simulink model "practice1_sim"  (R2020b)
settings: Solver=FixedStepAuto  StartTime=0.0  StopTime=simtime  FixedStep=step  RelTol=1e-3
undefined symbols (not defined in the file or in its folder): D, JL, JM, K, KE, KT, L, La, Ra
settings Model: Creator=yuto  LastModifiedBy=yuto

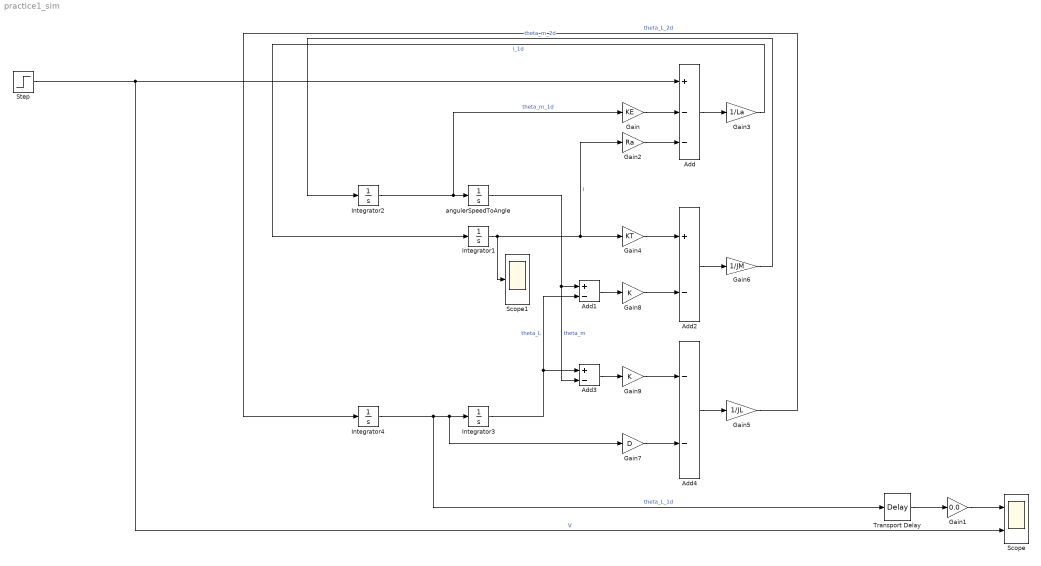
== system practice1_sim ==
  Add : Sum  Inputs=+--
  Add1 : Sum  Inputs=+-
  Add2 : Sum  Inputs=+-
  Add3 : Sum  Inputs=+-
  Add4 : Sum  Inputs=--
  Gain : Gain  Gain=KE
  Gain1 : Gain  Gain=0.0
  Gain2 : Gain  Gain=Ra
  Gain3 : Gain  Gain=1/La
  Gain4 : Gain  Gain=KT
  Gain5 : Gain  Gain=1/JL
  Gain6 : Gain  Gain=1/JM
  Gain7 : Gain  Gain=D
  Gain8 : Gain  Gain=K
  Gain9 : Gain  Gain=K
  Integrator{1..4} (4 alike) : Integrator
  Scope : Scope  NumInputPorts=2
  Scope1 : Scope
  Step : Step  Time=0  SampleTime=0
  Transport Delay : TransportDelay  DelayTime=L
  angulerSpeedToAngle : Integrator
  wires:
  angulerSpeedToAngle/1 -> Add3/2, Add1/1  "theta_m"
  Integrator2/1 -> Gain/1, angulerSpeedToAngle/1  "theta_m_1d"
  Integrator1/1 -> Scope1/1, Gain4/1, Gain2/1  "i"
  Gain3/1 -> Integrator1/1  "i_1d"
  Gain6/1 -> Integrator2/1  "theta_m_2d"
  Integrator4/1 -> Transport Delay/1, Gain7/1, Integrator3/1  "theta_L_1d"
  Gain5/1 -> Integrator4/1  "theta_L_2d"
  Step/1 -> Scope/2, Add/1  "V"
  Gain2/1 -> Add/3
  Gain/1 -> Add/2
  Add/1 -> Gain3/1
  Add1/1 -> Gain8/1
  Gain8/1 -> Add2/2
  Gain4/1 -> Add2/1
  Add2/1 -> Gain6/1
  Add3/1 -> Gain9/1
  Gain9/1 -> Add4/1
  Gain7/1 -> Add4/2
  Add4/1 -> Gain5/1
  Integrator3/1 -> Add1/2, Add3/1  "theta_L"
  Transport Delay/1 -> Gain1/1
  Gain1/1 -> Scope/1
